simulink model "motor_kit_sim_20MHz"  (R2024a)
settings: Solver=VariableStepAuto  StartTime=0.0  StopTime=10*62.5E-6  RelTol=1e-3  EnableMultiTasking=on
PreLoadFcn:
  | setup_motor_kit_sim_20MHz;
InitFcn:
  | setup_motor_kit_sim_20MHz;
values from neighbouring files (symbols this model uses):
  DSPBASampleTime = 0.05e-6    (= 5e-08)    [setup_motor_kit_sim_20MHz.m]
  wordLength = 16    [setup_motor_kit_sim_20MHz.m]
undefined symbols (not defined in the file or in its folder): AdvDSPBChannelOutDisplay, dpoly, dspba_internal_get_channel_ports, evalAionMaskParam, latency, primtype, value, x
libraries: DSPBAPrim x317, DSPBAModelBus x25, DSPBABase x7, dspsrcs4 x3, simulink x3, DSPBAUtilities x1
(part 3 of 4)

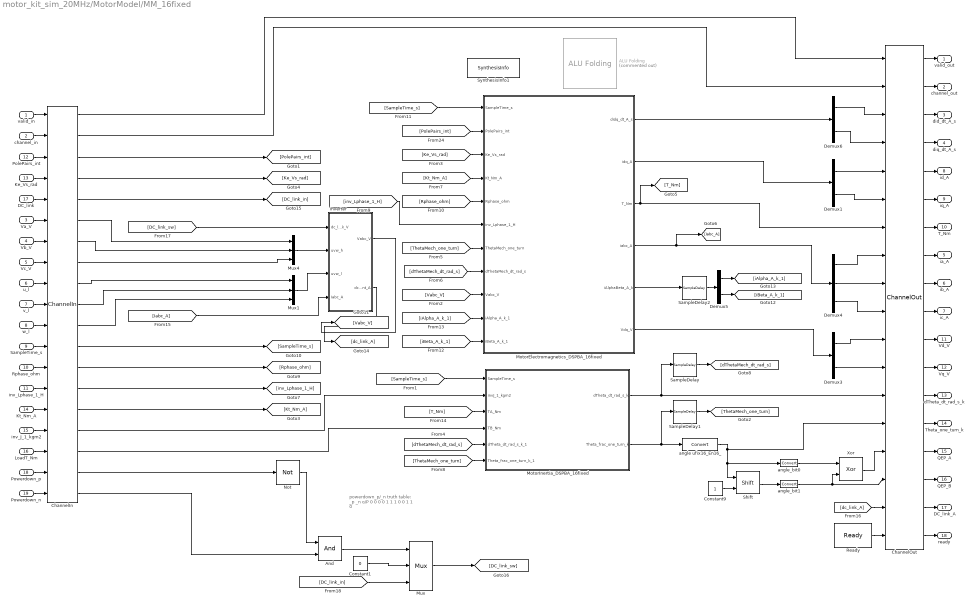
== system motor_kit_sim_20MHz/MotorModel/MM_16fixed ==
  note: powerdown_p/_n truth table:
      |
      | 	_p		_n		o/P
      | 	0		0		0
      | 	0		1		1
      | 	1		0		0
      | 	1		1		0
  valid_in : Inport
  channel_in : Inport  Port=2
  Va_V : Inport  Port=3
  Vb_V : Inport  Port=4
  Vc_V : Inport  Port=5
  u_l : Inport  Port=6  OutDataTypeStr=boolean
  v_l : Inport  Port=7  OutDataTypeStr=boolean
  w_l : Inport  Port=8  OutDataTypeStr=boolean
  SampleTime_s : Inport  Port=9
  Rphase_ohm : Inport  Port=10
  inv_Lphase_1_H : Inport  Port=11
  PolePairs_int : Inport  Port=12
  Ke_Vs_rad : Inport  Port=13
  Kt_Nm_A : Inport  Port=14
  inv_J_1_kgm2 : Inport  Port=15
  LoadT_Nm : Inport  Port=16
  DC_link : Inport  Port=17
  Powerdown_p : Inport  Port=18
  Powerdown_n : Inport  Port=19
  ALU Folding : DSPBAUtilities/ALU Folding  Description=Enables the new folder. When this block is placed in a subsystem, all primitive subsystems at the level it is placed and below will be passed to the folder. DSP Builder will then generate folded subsystems which can be placed back into the existing design.  Commented=on  version=20130913  genModelFileName=folded_model.xml  sampleRate=SampleRate  numChannels=1  maxLatency=LatencyConstraint  inputFormat=Parallel  outputFormat=Parallel  latchOutputs=off  originalRate=off  hasIdleState=off  padInputs=off  simRate=Data rate
  And : DSPBAPrim/And  primtype=and  nInputs=2  nOutputs=1  omode=Inherit via internal rule  otype=sfix(16)  scale=2^-15  rndmethod=Unbiased  factor=1  satmethod=Symmetric  shift_vec=[0 1 2 -1]  value=0  inPortNames=[' '; ' '; ' '; ' '; ' '; ' '; ' '; ' '; ' '; ' '; ' '; ' '; ' '; ' '; ' '; ' '; ]  outPortNames=[' ']  dspbaimage=dspba_prim.svg  text=fprintf('&');  version=20240716
  ChannelIn : DSPBAPrim/ChannelIn  primtype=channelin  nInputs=dspba_internal_get_channel_ports(gcb)  nOutputs=dspba_internal_get_channel_ports(gcb)  omode=Inherit via internal rule  otype=sfix(16)  scale=2^-15  rndmethod=Unbiased  factor=1  satmethod=Symmetric  shift_vec=[0 1 2 -1]  value=17  inPortNames=['v'; 'c'; '0'; '1'; '2'; '3'; '4'; '5'; '6'; '7'; '8'; '9'; 'A'; 'B'; 'D'; 'E'; 'F'; 'G'; 'H'; 'I'; 'J'; 'K'; 'L'; 'M'; 'N'; 'O'; 'P'; 'Q'; 'R'; 'S'; 'T'; 'U'; 'W'; 'X'; 'Y'; 'Z']  outPortNames=['v'; 'c'; '0'; '1'; '2'; '3'; '4'; '5'; '6'; '7'; '8'; '9'; 'A'; 'B'; 'D'; 'E'; 'F'; 'G'; 'H'; 'I'; 'J'; 'K'; 'L'; 'M'; 'N'; 'O'; 'P'; 'Q'; 'R'; 'S'; 'T'; 'U'; 'W'; 'X'; 'Y'; 'Z']  dspbaimage=dspba_prim_channel_tall.svg  text=fprintf('In');  dataSignals=17  foldingEnabled=off  packetBeginPresent=off  packetBeginEnabled=off  version=20231204
  ChannelOut : DSPBAPrim/ChannelOut  primtype=channelout  nInputs=dspba_internal_get_channel_ports(gcb)  nOutputs=dspba_internal_get_channel_ports(gcb)  omode=Inherit via internal rule  otype=sfix(16)  scale=2^-15  rndmethod=Unbiased  factor=1  satmethod=Symmetric  shift_vec=[0 1 2 -1]  value=16  inPortNames=['v'; 'c'; '0'; '1'; '2'; '3'; '4'; '5'; '6'; '7'; '8'; '9'; 'A'; 'B'; 'D'; 'E'; 'F'; 'G'; 'H'; 'I'; 'J'; 'K'; 'L'; 'M'; 'N'; 'O'; 'P'; 'Q'; 'R'; 'S'; 'T'; 'U'; 'W'; 'X'; 'Y'; 'Z']  outPortNames=['v'; 'c'; '0'; '1'; '2'; '3'; '4'; '5'; '6'; '7'; '8'; '9'; 'A'; 'B'; 'D'; 'E'; 'F'; 'G'; 'H'; 'I'; 'J'; 'K'; 'L'; 'M'; 'N'; 'O'; 'P'; 'Q'; 'R'; 'S'; 'T'; 'U'; 'W'; 'X'; 'Y'; 'Z']  dspbaimage=dspba_prim_channel_tall.svg  text=fprintf('Out%s', AdvDSPBChannelOutDisplay(latency));  dataSignals=16  foldingEnabled=off  packetBeginPresent=off  packetBeginEnabled=off  latency=53  version=20230901
  Constant1 : Constant  Value=0  OutDataTypeStr=fixdt(1,16,6)  SampleTime=DSPBASampleTime
  Constant9 : Constant  OutDataTypeStr=boolean
  Demux{1,3,5..6} (4 alike) : Demux  Outputs=2
  Demux4 : Demux  Outputs=3
  MotorElectromagnetics_DSPBA_16fixed : Subsystem
  MotorInertia_DSPBA_16fixed : Subsystem
  Mux : DSPBAPrim/Mux  primtype=mux  nInputs=evalAionMaskParam(gcb,'value',1)+1  nOutputs=1  omode=Inherit via internal rule  otype=sfix(16)  scale=2^-15  rndmethod=Unbiased  factor=1  satmethod=Symmetric  shift_vec=[0 1 2 -1]  value=2  inPortNames=['s '; 'd0'; 'd1'; 'd2'; 'd3'; 'd4'; 'd5'; 'd6'; 'd7'; 'd8'; 'd9';]  outPortNames=[' ']  dspbaimage=dspba_prim_tall.svg  text=fprintf('%s', primtype);  version=20240715
  Mux1 : Mux  Inputs=3
  Mux4 : Mux  Inputs=3
  Not : DSPBAPrim/Not  primtype=not  nInputs=1  nOutputs=1  omode=Inherit via internal rule  otype=sfix(16)  scale=2^-15  rndmethod=Unbiased  factor=1  satmethod=Symmetric  shift_vec=[0 1 2 -1]  value=0  inPortNames=[' '; ' ';]  outPortNames=[' ']  dspbaimage=dspba_prim.svg  text=fprintf('~');  version=20240716
  Ready : DSPBAPrim/Ready  primtype=ready  nInputs=0  nOutputs=1  omode=Inherit via internal rule  otype=ufix(1)  scale=2^-0  rndmethod=Unbiased  factor=1  satmethod=Asymmetric  shift_vec=[]  value=1  inPortNames=['']  outPortNames=[' ']  dspbaimage=dspba_prim.svg  text=fprintf('Ready');  version=20240719
  SampleDelay : DSPBAPrim/SampleDelay  primtype=sampdelay  nInputs=1  nOutputs=1  omode=Inherit via internal rule  otype=sfix(16)  scale=2^-15  floatPrecision=float32_m23  rndmethod=Unbiased  factor=1  satmethod=Symmetric  shift_vec=[0 1 2 -1]  value=25  inPortNames=[' '; ' ';]  outPortNames=[' ']  dspbaimage=dspba_prim.svg  text=dpoly(1, eye(1,value+1), 'z')  flexible=on  slackgroup=0  augmented=28  version=20240711  advOptions=[]
  SampleDelay1 : DSPBAPrim/SampleDelay  primtype=sampdelay  nInputs=1  nOutputs=1  omode=Inherit via internal rule  otype=sfix(16)  scale=2^-15  floatPrecision=float32_m23  rndmethod=Unbiased  factor=1  satmethod=Symmetric  shift_vec=[0 1 2 -1]  value=33  inPortNames=[' '; ' ';]  outPortNames=[' ']  dspbaimage=dspba_prim.svg  text=dpoly(1, eye(1,value+1), 'z')  flexible=on  slackgroup=0  augmented=28  version=20240711  advOptions=[]
  SampleDelay2 : DSPBAPrim/SampleDelay  primtype=sampdelay  nInputs=1  nOutputs=1  omode=Inherit via internal rule  otype=sfix(16)  scale=2^-15  floatPrecision=float32_m23  rndmethod=Unbiased  factor=1  satmethod=Symmetric  shift_vec=[0 1 2 -1]  value=1  inPortNames=[' '; ' ';]  outPortNames=[' ']  dspbaimage=dspba_prim.svg  text=dpoly(1, eye(1,value+1), 'z')  flexible=off  slackgroup=0  augmented=0  version=20240711  advOptions=[]
  Shift : DSPBAPrim/Shift  primtype=shift  nInputs=2  nOutputs=1  omode=Specify via dialog  otype=ufix(16)  scale=2^-16  rndmethod=Unbiased  factor=1  satmethod=Symmetric  shift_vec=[0 1 2 -1]  value=0  inPortNames=['a'; 'b';]  outPortNames=[' ']  dspbaimage=dspba_prim.svg  text=fprintf('a >> b');  version=20240716
  SynthesisInfo1 : DSPBAPrim/SynthesisInfo  primtype=synthinfo  nInputs=0  nOutputs=0  omode=Inherit via internal rule  otype=sfix(16)  scale=2^-15  rndmethod=Truncate  factor=1  satmethod=Symmetric  shift_vec=[0 1 2 -1]  value=99  inPortNames=[' '; ' ';]  outPortNames=[' ']  dspbaimage=dspba_prim_ctrl.jpg  text=fprintf('Style=%s', style);  style=Scheduled  constraintPair=None  constraintRelation=>  constraintLimit=2  modelRefSign=+  modelRef=''  showSchedule=off  simulationMode=Use Global Value  resetMinimization=Conditional - On for ChannelIn/Out only  version=20230821
  Xor : DSPBAPrim/Xor  primtype=xor  nInputs=2  nOutputs=1  omode=Inherit via internal rule  otype=sfix(16)  scale=2^-15  rndmethod=Unbiased  factor=1  satmethod=Symmetric  shift_vec=[0 1 2 -1]  value=0  inPortNames=[' '; ' '; ' '; ' '; ' '; ' '; ' '; ' '; ' '; ' '; ' '; ' '; ' '; ' '; ' '; ' '; ]  outPortNames=[' ']  dspbaimage=dspba_prim.svg  text=fprintf('^');  version=20240716
  angle ufix16_En16_ : DSPBAPrim/Convert  primtype=convert  nInputs=1  nOutputs=1  omode=Specify via dialog  otype=ufix(16)  scale=2^-16  floatPrecision=float32_m23  rndmethod=Unbiased  factor=1  satmethod=None  shift_vec=[0 1 2 -1]  value=round([0:255]/17)  inPortNames=[' '; ' ';]  outPortNames=[' '; 'c']  dspbaimage=dspba_prim_wide.svg  text=fprintf('convert');  clipdetect=off  advOptions=[]  version=20240711
  angle_bit0 : DSPBAPrim/Convert  primtype=convert  nInputs=1  nOutputs=1  omode=Specify via dialog  otype=ufix(1)  scale=2^-13  floatPrecision=float32_m23  rndmethod=Truncate  factor=1  satmethod=None  shift_vec=[0 1 2 -1]  value=round([0:255]/17)  inPortNames=[' '; ' ';]  outPortNames=[' '; 'c']  dspbaimage=dspba_prim_wide.svg  text=fprintf('convert');  clipdetect=off  advOptions=[]  version=20240711
  angle_bit1 : DSPBAPrim/Convert  primtype=convert  nInputs=1  nOutputs=1  omode=Specify via dialog  otype=ufix(1)  scale=2^-13  floatPrecision=float32_m23  rndmethod=Truncate  factor=1  satmethod=None  shift_vec=[0 1 2 -1]  value=round([0:255]/17)  inPortNames=[' '; ' ';]  outPortNames=[' '; 'c']  dspbaimage=dspba_prim_wide.svg  text=fprintf('convert');  clipdetect=off  advOptions=[]  version=20240711
  inverter : Subsystem
  valid_out : Outport
  channel_out : Outport  Port=2
  did_dt_A_s : Outport  Port=3
  diq_dt_A_s : Outport  Port=4
  ia_A : Outport  Port=5
  ib_A : Outport  Port=6
  ic_A : Outport  Port=7
  id_A : Outport  Port=8
  iq_A : Outport  Port=9
  T_Nm : Outport  Port=10
  Vd_V : Outport  Port=11
  Vq_V : Outport  Port=12
  dTheta_dt_rad_s_k : Outport  Port=13
  Theta_one_turn_k : Outport  Port=14
  QEP_A : Outport  Port=15
  QEP_B : Outport  Port=16
  DC_link_A : Outport  Port=17
  ready : Outport  Port=18
  wires:
  [SampleTime_s] -> MotorElectromagnetics_DSPBA_16fixed/1(SampleTime_s)
  [PolePairs_int] -> MotorElectromagnetics_DSPBA_16fixed/2(PolePairs_int)
  [Ke_Vs_rad] -> MotorElectromagnetics_DSPBA_16fixed/3(Ke_Vs_rad)
  [Kt_Nm_A] -> MotorElectromagnetics_DSPBA_16fixed/4(Kt_Nm_A)
  [Rphase_ohm] -> MotorElectromagnetics_DSPBA_16fixed/5(Rphase_ohm)
  [inv_Lphase_1_H] -> MotorElectromagnetics_DSPBA_16fixed/6(inv_Lphase_1_H)
  [Vabc_V] -> MotorElectromagnetics_DSPBA_16fixed/9(Vabc_V)
  [iAlpha_A_k_1] -> MotorElectromagnetics_DSPBA_16fixed/10(iAlpha_A_k_1)
  [iBeta_A_k_1] -> MotorElectromagnetics_DSPBA_16fixed/11(iBeta_A_k_1)
  MotorElectromagnetics_DSPBA_16fixed/1(didq_dt_A_s) -> Demux6/1
  MotorElectromagnetics_DSPBA_16fixed/2(idq_A) -> Demux1/1
  MotorElectromagnetics_DSPBA_16fixed/3(T_Nm) -> ChannelOut/7, [T_Nm]
  [SampleTime_s] -> MotorInertia_DSPBA_16fixed/1(SampleTime_s)
  [dThetaMech_dt_rad_s] -> MotorInertia_DSPBA_16fixed/5(dTheta_dt_rad_s_k_1)
  [ThetaMech_one_turn] -> MotorInertia_DSPBA_16fixed/6(Theta_frac_one_turn_k_1)
  [T_Nm] -> MotorInertia_DSPBA_16fixed/3(TA_Nm)
  valid_in/1 -> ChannelIn/1
  channel_in/1 -> ChannelIn/2
  PolePairs_int/1 -> ChannelIn/3
  ChannelOut/1 -> valid_out/1
  ChannelOut/3 -> did_dt_A_s/1
  ChannelOut/2 -> channel_out/1
  ChannelOut/4 -> diq_dt_A_s/1
  ChannelOut/5 -> id_A/1
  ChannelOut/6 -> iq_A/1
  ChannelOut/7 -> T_Nm/1
  ChannelOut/8 -> ia_A/1
  ChannelOut/9 -> ib_A/1
  ChannelOut/10 -> ic_A/1
  ChannelIn/1 -> ChannelOut/1
  ChannelIn/2 -> ChannelOut/2
  ChannelIn/3 -> [PolePairs_int]
  Demux6/1 -> ChannelOut/3
  Demux6/2 -> ChannelOut/4
  Demux1/1 -> ChannelOut/5
  Demux1/2 -> ChannelOut/6
  MotorElectromagnetics_DSPBA_16fixed/4(iabc_A) -> [Iabc_A], Demux4/1
  Demux4/1 -> ChannelOut/8
  Demux4/2 -> ChannelOut/9
  Demux4/3 -> ChannelOut/10
  MotorElectromagnetics_DSPBA_16fixed/5(iAlphaBeta_A_k) -> SampleDelay2/1
  MotorElectromagnetics_DSPBA_16fixed/6(Vdq_V) -> Demux3/1
  MotorInertia_DSPBA_16fixed/1(dTheta_dt_rad_s_k) -> SampleDelay/1, ChannelOut/13
  SampleDelay1/1 -> [ThetaMech_one_turn]
  [ThetaMech_one_turn] -> MotorElectromagnetics_DSPBA_16fixed/7(ThetaMech_one_turn)
  [dThetaMech_dt_rad_s] -> MotorElectromagnetics_DSPBA_16fixed/8(dThetaMech_dt_rad_s)
  SampleDelay/1 -> [dThetaMech_dt_rad_s]
  SampleDelay2/1 -> Demux5/1
  Demux5/1 -> [iAlpha_A_k_1]
  Demux5/2 -> [iBeta_A_k_1]
  Ke_Vs_rad/1 -> ChannelIn/4
  ChannelIn/8 -> Mux4/3
  ChannelIn/6 -> Mux4/1
  ChannelIn/4 -> [Ke_Vs_rad]
  ChannelIn/7 -> Mux4/2
  Demux3/1 -> ChannelOut/11
  Demux3/2 -> ChannelOut/12
  ChannelOut/11 -> Vd_V/1
  ChannelOut/12 -> Vq_V/1
  ChannelOut/13 -> dTheta_dt_rad_s_k/1
  ChannelOut/14 -> Theta_one_turn_k/1
  Vc_V/1 -> ChannelIn/8
  Vb_V/1 -> ChannelIn/7
  Va_V/1 -> ChannelIn/6
  DC_link/1 -> ChannelIn/5
  Constant9/1 -> Shift/2
  Xor/1 -> ChannelOut/15
  Shift/1 -> angle_bit1/1
  angle_bit1/1 -> ChannelOut/16, Xor/2
  MotorInertia_DSPBA_16fixed/2(Theta_frac_one_turn_k) -> angle ufix16_En16_/1, SampleDelay1/1
  angle_bit0/1 -> Xor/1
  ChannelOut/15 -> QEP_A/1
  ChannelOut/16 -> QEP_B/1
  angle ufix16_En16_/1 -> ChannelOut/14, Shift/1, angle_bit0/1
  ChannelIn/5 -> [DC_link_in]
  u_l/1 -> ChannelIn/9
  w_l/1 -> ChannelIn/11
  v_l/1 -> ChannelIn/10
  SampleTime_s/1 -> ChannelIn/12
  Rphase_ohm/1 -> ChannelIn/13
  inv_Lphase_1_H/1 -> ChannelIn/14
  Kt_Nm_A/1 -> ChannelIn/15
  inv_J_1_kgm2/1 -> ChannelIn/16
  LoadT_Nm/1 -> ChannelIn/17
  ChannelIn/17 -> MotorInertia_DSPBA_16fixed/4(TB_Nm)
  ChannelIn/16 -> MotorInertia_DSPBA_16fixed/2(invJ_1_kgm2)
  ChannelIn/12 -> [SampleTime_s]
  ChannelIn/13 -> [Rphase_ohm]
  ChannelIn/15 -> [Kt_Nm_A]
  ChannelIn/14 -> [inv_Lphase_1_H]
  Mux1/1 -> inverter/3(uvw_l)
  ChannelIn/9 -> Mux1/1
  ChannelIn/11 -> Mux1/3
  ChannelIn/10 -> Mux1/2
  Mux4/1 -> inverter/2(uvw_h)
  inverter/1(Vabc_V) -> [Vabc_V]
  [Iabc_A] -> inverter/4(Iabc_A)
  Ready/1 -> ChannelOut/18
  ChannelOut/17 -> DC_link_A/1
  ChannelOut/18 -> ready/1
  [dc_link_A] -> ChannelOut/17
  inverter/2(dc_link_current_A) -> [dc_link_A]
  [DC_link_sw] -> inverter/1(dc_link_V)
  [DC_link_in] -> Mux/3
  Mux/1 -> [DC_link_sw]
  Constant1/1 -> Mux/2
  Not/1 -> And/1
  And/1 -> Mux/1
  Powerdown_p/1 -> ChannelIn/18
  Powerdown_n/1 -> ChannelIn/19
  ChannelIn/18 -> Not/1
  ChannelIn/19 -> And/2

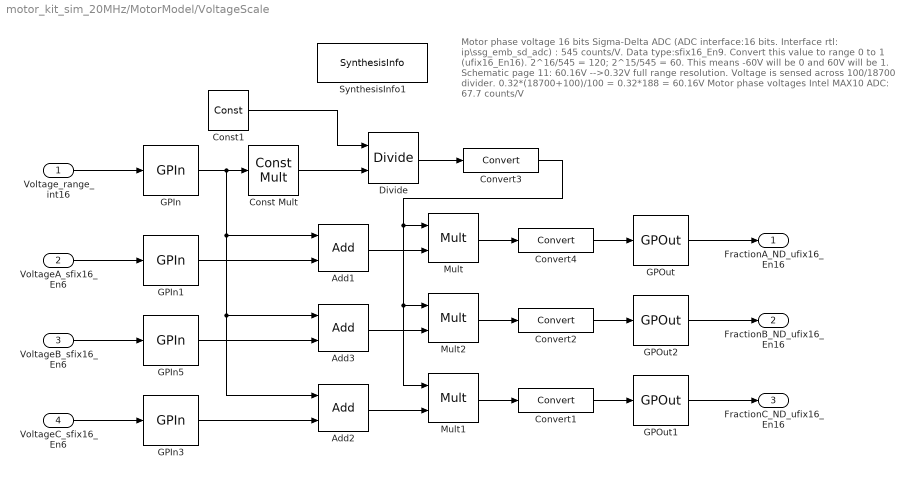
== system motor_kit_sim_20MHz/MotorModel/VoltageScale ==
  note: Motor phase voltage 16 bits Sigma-Delta ADC (ADC interface:16 bits. Interface rtl: ip\ssg_emb_sd_adc) : 545 counts/V. Data type:sfix16_En9. Convert this value to range 0 to 1 (ufix16_En16). 2^16/545 = 120; 2^15/545 = 60. This means -60V will be 0 and 60V will be 1.
      | Schematic page 11: 60.16V -->0.32V full range resolution. Voltage is sensed across 100/18700 divider. 0.32*(18700+100)/100 = 0.32*188 = 60.16V
      | Motor phase voltages Intel MAX10 ADC: 67.7 counts/V
  Voltage_range_int16 : Inport
  VoltageA_sfix16_En6 : Inport  Port=2
  VoltageB_sfix16_En6 : Inport  Port=3
  VoltageC_sfix16_En6 : Inport  Port=4
  Add1 : DSPBAPrim/Add  primtype=add  nInputs=evalAionMaskParam(gcb,'value',1)  nOutputs=1  omode=Inherit via internal rule with word growth  otype=sfix(16)  scale=2^-15  rndmethod=Unbiased  factor=1  satmethod=Symmetric  shift_vec=[0 1 2 -1]  value=2  inPortNames=[' '; ' ';]  outPortNames=[' ']  dspbaimage=dspba_prim.svg  text=fprintf('+');  genFPC=off  floatRounding=correct  advOptions=[]  version=20240716
  Add2 : DSPBAPrim/Add  primtype=add  nInputs=evalAionMaskParam(gcb,'value',1)  nOutputs=1  omode=Inherit via internal rule with word growth  otype=sfix(16)  scale=2^-15  rndmethod=Unbiased  factor=1  satmethod=Symmetric  shift_vec=[0 1 2 -1]  value=2  inPortNames=[' '; ' ';]  outPortNames=[' ']  dspbaimage=dspba_prim.svg  text=fprintf('+');  genFPC=off  floatRounding=correct  advOptions=[]  version=20240716
  Add3 : DSPBAPrim/Add  primtype=add  nInputs=evalAionMaskParam(gcb,'value',1)  nOutputs=1  omode=Inherit via internal rule with word growth  otype=sfix(16)  scale=2^-15  rndmethod=Unbiased  factor=1  satmethod=Symmetric  shift_vec=[0 1 2 -1]  value=2  inPortNames=[' '; ' ';]  outPortNames=[' ']  dspbaimage=dspba_prim.svg  text=fprintf('+');  genFPC=off  floatRounding=correct  advOptions=[]  version=20240716
  Const Mult : DSPBAPrim/Const Mult  primtype=constmult  nInputs=1  nOutputs=1  omode=Inherit via internal rule  otype=sfix(16)  scale=2^-15  rndmethod=Unbiased  factor=1  satmethod=Symmetric  shift_vec=[0 1 2 -1]  value=2  inPortNames=[' '; ' ';]  outPortNames=[' ']  dspbaimage=dspba_prim.svg  text=fprintf('cx');  floatRounding=correct  advOptions=[]  version=20240716
  Const1 : DSPBAPrim/Const  primtype=const  nInputs=0  nOutputs=1  omode=Specify via dialog  otype=sfix(2)  scale=1  floatPrecision=float32_m23  rndmethod=Unbiased  factor=1  satmethod=Symmetric  shift_vec=[0 1 2 -1]  value=1  inPortNames=['+'; '+';]  outPortNames=[' ']  dspbaimage=dspba_prim.svg  text=fprintf('%s', num2str(value));  warnSaturation=on  version=20240711  SampleTime=inf
  Convert1 : DSPBAPrim/Convert  primtype=convert  nInputs=1  nOutputs=1  omode=Specify via dialog  otype=DataTypeFraction  scale=constScaleFraction  floatPrecision=float32_m23  rndmethod=Biased  factor=1  satmethod=None  shift_vec=[0 1 2 -1]  value=round([0:255]/17)  inPortNames=[' '; ' ';]  outPortNames=[' '; 'c']  dspbaimage=dspba_prim_wide.svg  text=fprintf('convert');  clipdetect=off  advOptions=[]  version=20240711
  Convert2 : DSPBAPrim/Convert  primtype=convert  nInputs=1  nOutputs=1  omode=Specify via dialog  otype=DataTypeFraction  scale=constScaleFraction  floatPrecision=float32_m23  rndmethod=Biased  factor=1  satmethod=None  shift_vec=[0 1 2 -1]  value=round([0:255]/17)  inPortNames=[' '; ' ';]  outPortNames=[' '; 'c']  dspbaimage=dspba_prim_wide.svg  text=fprintf('convert');  clipdetect=off  advOptions=[]  version=20240711
  Convert3 : DSPBAPrim/Convert  primtype=convert  nInputs=1  nOutputs=1  omode=Specify via dialog  otype=sfix(18)  scale=constScaleFraction  floatPrecision=float32_m23  rndmethod=Biased  factor=1  satmethod=None  shift_vec=[0 1 2 -1]  value=round([0:255]/17)  inPortNames=[' '; ' ';]  outPortNames=[' '; 'c']  dspbaimage=dspba_prim_wide.svg  text=fprintf('convert');  clipdetect=off  advOptions=[]  version=20240711
  Convert4 : DSPBAPrim/Convert  primtype=convert  nInputs=1  nOutputs=1  omode=Specify via dialog  otype=DataTypeFraction  scale=constScaleFraction  floatPrecision=float32_m23  rndmethod=Biased  factor=1  satmethod=None  shift_vec=[0 1 2 -1]  value=round([0:255]/17)  inPortNames=[' '; ' ';]  outPortNames=[' '; 'c']  dspbaimage=dspba_prim_wide.svg  text=fprintf('convert');  clipdetect=off  advOptions=[]  version=20240711
  Divide : DSPBAPrim/Divide  primtype=divide  nInputs=2  nOutputs=1  omode=Inherit via internal rule  otype=sfix(16)  scale=2^-15  rndmethod=Unbiased  factor=1  satmethod=Symmetric  shift_vec=[0 1 2 -1]  value=round([0:255]/17)  inPortNames=[' '; ' ';]  outPortNames=[' ']  dspbaimage=dspba_prim.svg  text=fprintf('a\n----\nb');  floatRounding=correct  intDivider=off  advOptions=[]  version=20240716
  GPIn{,1,3,5} (4 alike) : DSPBAPrim/GPIn  primtype=gpin  nInputs=evalAionMaskParam(gcb,'value',1)  nOutputs=evalAionMaskParam(gcb,'value',1)  omode=Inherit via internal rule  otype=sfix(16)  scale=2^-15  rndmethod=Unbiased  factor=1  satmethod=Symmetric  shift_vec=[0 1 2 -1]  value=1  inPortNames=[' ' ' ' ' ' ' ' ' ' ' ' ' ' ' ' ' ' ' ' ' ' ' ' ' ' ' ' ' ' ' ' ' ' ' ' ' ' ' ' ' ' ' ' ' ' ' ' ' ' ' ' ' ' ' ' ' ' ' ' ' ' ' ' ' ' ' ' ' ']'  outPortNames=[' ' ' ' ' ' ' ' ' ' ' ' ' ' ' ' ' ' ' ' ' ' ' ' ' ' ' ' ' ' ' ' ' ' ' ' ' ' ' ' ' ' ' ' ' ' ' ' ' ' ' ' ' ' ' ' ' ' ' ' ' ' ' ' ' ' ' ' ' ']'  dspbaimage=dspba_prim_channel_tall.svg  text=fprintf('GPIn');  version=20231204
  GPOut : DSPBAPrim/GPOut  primtype=gpout  nInputs=evalAionMaskParam(gcb,'value',1)  nOutputs=evalAionMaskParam(gcb,'value',1)  omode=Inherit via internal rule  otype=sfix(16)  scale=2^-15  rndmethod=Unbiased  factor=1  satmethod=Symmetric  shift_vec=[0 1 2 -1]  value=1  inPortNames=[' ' ' ' ' ' ' ' ' ' ' ' ' ' ' ' ' ' ' ' ' ' ' ' ' ' ' ' ' ' ' ' ' ' ' ' ' ' ' ' ' ' ' ' ' ' ' ' ' ' ' ' ' ' ' ' ' ' ' ' ' ' ' ' ' ' ' ' ' ']'  outPortNames=[' ' ' ' ' ' ' ' ' ' ' ' ' ' ' ' ' ' ' ' ' ' ' ' ' ' ' ' ' ' ' ' ' ' ' ' ' ' ' ' ' ' ' ' ' ' ' ' ' ' ' ' ' ' ' ' ' ' ' ' ' ' ' ' ' ' ' ' ' ']'  dspbaimage=dspba_prim_channel_tall.svg  text=fprintf('GPOut');  latency=21  version=20230904
  GPOut1 : DSPBAPrim/GPOut  primtype=gpout  nInputs=evalAionMaskParam(gcb,'value',1)  nOutputs=evalAionMaskParam(gcb,'value',1)  omode=Inherit via internal rule  otype=sfix(16)  scale=2^-15  rndmethod=Unbiased  factor=1  satmethod=Symmetric  shift_vec=[0 1 2 -1]  value=1  inPortNames=[' ' ' ' ' ' ' ' ' ' ' ' ' ' ' ' ' ' ' ' ' ' ' ' ' ' ' ' ' ' ' ' ' ' ' ' ' ' ' ' ' ' ' ' ' ' ' ' ' ' ' ' ' ' ' ' ' ' ' ' ' ' ' ' ' ' ' ' ' ']'  outPortNames=[' ' ' ' ' ' ' ' ' ' ' ' ' ' ' ' ' ' ' ' ' ' ' ' ' ' ' ' ' ' ' ' ' ' ' ' ' ' ' ' ' ' ' ' ' ' ' ' ' ' ' ' ' ' ' ' ' ' ' ' ' ' ' ' ' ' ' ' ' ']'  dspbaimage=dspba_prim_channel_tall.svg  text=fprintf('GPOut');  latency=21  version=20230904
  GPOut2 : DSPBAPrim/GPOut  primtype=gpout  nInputs=evalAionMaskParam(gcb,'value',1)  nOutputs=evalAionMaskParam(gcb,'value',1)  omode=Inherit via internal rule  otype=sfix(16)  scale=2^-15  rndmethod=Unbiased  factor=1  satmethod=Symmetric  shift_vec=[0 1 2 -1]  value=1  inPortNames=[' ' ' ' ' ' ' ' ' ' ' ' ' ' ' ' ' ' ' ' ' ' ' ' ' ' ' ' ' ' ' ' ' ' ' ' ' ' ' ' ' ' ' ' ' ' ' ' ' ' ' ' ' ' ' ' ' ' ' ' ' ' ' ' ' ' ' ' ' ']'  outPortNames=[' ' ' ' ' ' ' ' ' ' ' ' ' ' ' ' ' ' ' ' ' ' ' ' ' ' ' ' ' ' ' ' ' ' ' ' ' ' ' ' ' ' ' ' ' ' ' ' ' ' ' ' ' ' ' ' ' ' ' ' ' ' ' ' ' ' ' ' ' ']'  dspbaimage=dspba_prim_channel_tall.svg  text=fprintf('GPOut');  latency=21  version=20230904
  Mult : DSPBAPrim/Mult  primtype=mult  nInputs=2  nOutputs=1  omode=Inherit via internal rule  otype=sfix(16)  scale=2^-15  floatPrecision=float32_m23  rndmethod=Unbiased  factor=1  satmethod=Symmetric  shift_vec=[0 1 2 -1]  value=0  inPortNames=[' '; ' ';]  outPortNames=[' ']  dspbaimage=dspba_prim.svg  text=fprintf('X');  floatRounding=correct  advOptions=[]  version=20240711
  Mult1 : DSPBAPrim/Mult  primtype=mult  nInputs=2  nOutputs=1  omode=Inherit via internal rule  otype=sfix(16)  scale=2^-15  floatPrecision=float32_m23  rndmethod=Unbiased  factor=1  satmethod=Symmetric  shift_vec=[0 1 2 -1]  value=0  inPortNames=[' '; ' ';]  outPortNames=[' ']  dspbaimage=dspba_prim.svg  text=fprintf('X');  floatRounding=correct  advOptions=[]  version=20240711
  Mult2 : DSPBAPrim/Mult  primtype=mult  nInputs=2  nOutputs=1  omode=Inherit via internal rule  otype=sfix(16)  scale=2^-15  floatPrecision=float32_m23  rndmethod=Unbiased  factor=1  satmethod=Symmetric  shift_vec=[0 1 2 -1]  value=0  inPortNames=[' '; ' ';]  outPortNames=[' ']  dspbaimage=dspba_prim.svg  text=fprintf('X');  floatRounding=correct  advOptions=[]  version=20240711
  SynthesisInfo1 : DSPBAPrim/SynthesisInfo  primtype=synthinfo  nInputs=0  nOutputs=0  omode=Inherit via internal rule  otype=sfix(16)  scale=2^-15  rndmethod=Truncate  factor=1  satmethod=Symmetric  shift_vec=[0 1 2 -1]  value=99  inPortNames=[' '; ' ';]  outPortNames=[' ']  dspbaimage=dspba_prim_ctrl.jpg  text=fprintf('Style=%s', style);  style=Scheduled  constraintPair=None  constraintRelation=>  constraintLimit=2  modelRefSign=+  modelRef=''  showSchedule=off  simulationMode=Use Global Value  resetMinimization=Conditional - On for ChannelIn/Out only  version=20230821
  "FractionA_ND_ufix16_En16 " : Outport
  FractionB_ND_ufix16_En16 : Outport  Port=2
  FractionC_ND_ufix16_En16 : Outport  Port=3
  wires:
  GPOut2/1 -> FractionB_ND_ufix16_En16/1
  GPOut1/1 -> FractionC_ND_ufix16_En16/1
  Convert2/1 -> GPOut2/1
  Convert1/1 -> GPOut1/1
  Mult1/1 -> Convert1/1
  Mult/1 -> Convert4/1
  Const1/1 -> Divide/1
  VoltageC_sfix16_En6/1 -> GPIn3/1
  Mult2/1 -> Convert2/1
  Voltage_range_int16/1 -> GPIn/1
  VoltageB_sfix16_En6/1 -> GPIn5/1
  GPOut/1 -> "FractionA_ND_ufix16_En16 "/1
  GPIn/1 -> Const Mult/1, Add1/1, Add3/1, Add2/1
  GPIn3/1 -> Add2/2
  Convert4/1 -> GPOut/1
  GPIn5/1 -> Add3/2
  VoltageA_sfix16_En6/1 -> GPIn1/1
  Add2/1 -> Mult1/2
  Add3/1 -> Mult2/2
  Add1/1 -> Mult/2
  GPIn1/1 -> Add1/2
  Const Mult/1 -> Divide/2
  Divide/1 -> Convert3/1
  Convert3/1 -> Mult1/1, Mult2/1, Mult/1

== system motor_kit_sim_20MHz/MotorModel/Voltage_scale_120_link_V ==
  note: DC link voltage 16 bits Sigma-Delta ADC (ADC interface:16 bits. Interface rtl: ip\dspba\two_phase_dc_dc\rtl\psg_ecfs_lvdcdc_sd_adc\hdl) : 545 counts/V. Data type:sfix16_En9. Convert this value to range 0 to 1 (ufix16_En16). 2^16/545 = 120; 2^15/545 = 60. This means -60V will be 0 and 60V will be 1.
      | Schematic page 6: 60.16V -->0.32V full range resolution. Voltage is sensed across 100/18700 divider. 0.32*(18700+100)/100=60.16V
      | This voltage has been scaled differently to be feedback into DC-DC controller IP.
      | Scaling for DC-DC controller IP input voltage_fdbk: 40 counts/V. This scaling is handled within ip\dspba\two_phase_dc_dc\rtl\psg_ecfs_lvdcdc_sd_adc\hdl\psg_ecfs_lvdcdc_sd_adc.v, it is scaled in hardware.
      | DC link voltage Intel MAX10 ADC: 67.7 counts/V
  Voltage_range_int16 : Inport
  Voltage_sfix16_En9 : Inport  Port=2
  Add1 : DSPBAPrim/Add  primtype=add  nInputs=evalAionMaskParam(gcb,'value',1)  nOutputs=1  omode=Inherit via internal rule with word growth  otype=sfix(16)  scale=2^-15  rndmethod=Unbiased  factor=1  satmethod=Symmetric  shift_vec=[0 1 2 -1]  value=2  inPortNames=[' '; ' ';]  outPortNames=[' ']  dspbaimage=dspba_prim.svg  text=fprintf('+');  genFPC=off  floatRounding=correct  advOptions=[]  version=20240716
  Const2 : DSPBAPrim/Const  primtype=const  nInputs=0  nOutputs=1  omode=Specify via dialog  otype=DataType  scale=constScaleFraction  floatPrecision=float32_m23  rndmethod=Unbiased  factor=1  satmethod=Symmetric  shift_vec=[0 1 2 -1]  value=1/2  inPortNames=['+'; '+';]  outPortNames=[' ']  dspbaimage=dspba_prim.svg  text=fprintf('%s', num2str(value));  warnSaturation=on  version=20240711  SampleTime=inf
  Convert4 : DSPBAPrim/Convert  primtype=convert  nInputs=1  nOutputs=1  omode=Specify via dialog  otype=DataTypeFraction  scale=constScaleFraction  floatPrecision=float32_m23  rndmethod=Biased  factor=1  satmethod=None  shift_vec=[0 1 2 -1]  value=round([0:255]/17)  inPortNames=[' '; ' ';]  outPortNames=[' '; 'c']  dspbaimage=dspba_prim_wide.svg  text=fprintf('convert');  clipdetect=off  advOptions=[]  version=20240711
  Divide : DSPBAPrim/Divide  primtype=divide  nInputs=2  nOutputs=1  omode=Inherit via internal rule  otype=sfix(16)  scale=2^-15  rndmethod=Unbiased  factor=1  satmethod=Symmetric  shift_vec=[0 1 2 -1]  value=round([0:255]/17)  inPortNames=[' '; ' ';]  outPortNames=[' ']  dspbaimage=dspba_prim.svg  text=fprintf('a\n----\nb');  floatRounding=correct  intDivider=off  advOptions=[]  version=20240716
  GPIn : DSPBAPrim/GPIn  primtype=gpin  nInputs=evalAionMaskParam(gcb,'value',1)  nOutputs=evalAionMaskParam(gcb,'value',1)  omode=Inherit via internal rule  otype=sfix(16)  scale=2^-15  rndmethod=Unbiased  factor=1  satmethod=Symmetric  shift_vec=[0 1 2 -1]  value=1  inPortNames=[' ' ' ' ' ' ' ' ' ' ' ' ' ' ' ' ' ' ' ' ' ' ' ' ' ' ' ' ' ' ' ' ' ' ' ' ' ' ' ' ' ' ' ' ' ' ' ' ' ' ' ' ' ' ' ' ' ' ' ' ' ' ' ' ' ' ' ' ' ']'  outPortNames=[' ' ' ' ' ' ' ' ' ' ' ' ' ' ' ' ' ' ' ' ' ' ' ' ' ' ' ' ' ' ' ' ' ' ' ' ' ' ' ' ' ' ' ' ' ' ' ' ' ' ' ' ' ' ' ' ' ' ' ' ' ' ' ' ' ' ' ' ' ']'  dspbaimage=dspba_prim_channel_tall.svg  text=fprintf('GPIn');  version=20231204
  GPIn1 : DSPBAPrim/GPIn  primtype=gpin  nInputs=evalAionMaskParam(gcb,'value',1)  nOutputs=evalAionMaskParam(gcb,'value',1)  omode=Inherit via internal rule  otype=sfix(16)  scale=2^-15  rndmethod=Unbiased  factor=1  satmethod=Symmetric  shift_vec=[0 1 2 -1]  value=1  inPortNames=[' ' ' ' ' ' ' ' ' ' ' ' ' ' ' ' ' ' ' ' ' ' ' ' ' ' ' ' ' ' ' ' ' ' ' ' ' ' ' ' ' ' ' ' ' ' ' ' ' ' ' ' ' ' ' ' ' ' ' ' ' ' ' ' ' ' ' ' ' ']'  outPortNames=[' ' ' ' ' ' ' ' ' ' ' ' ' ' ' ' ' ' ' ' ' ' ' ' ' ' ' ' ' ' ' ' ' ' ' ' ' ' ' ' ' ' ' ' ' ' ' ' ' ' ' ' ' ' ' ' ' ' ' ' ' ' ' ' ' ' ' ' ' ']'  dspbaimage=dspba_prim_channel_tall.svg  text=fprintf('GPIn');  version=20231204
  GPOut : DSPBAPrim/GPOut  primtype=gpout  nInputs=evalAionMaskParam(gcb,'value',1)  nOutputs=evalAionMaskParam(gcb,'value',1)  omode=Inherit via internal rule  otype=sfix(16)  scale=2^-15  rndmethod=Unbiased  factor=1  satmethod=Symmetric  shift_vec=[0 1 2 -1]  value=1  inPortNames=[' ' ' ' ' ' ' ' ' ' ' ' ' ' ' ' ' ' ' ' ' ' ' ' ' ' ' ' ' ' ' ' ' ' ' ' ' ' ' ' ' ' ' ' ' ' ' ' ' ' ' ' ' ' ' ' ' ' ' ' ' ' ' ' ' ' ' ' ' ']'  outPortNames=[' ' ' ' ' ' ' ' ' ' ' ' ' ' ' ' ' ' ' ' ' ' ' ' ' ' ' ' ' ' ' ' ' ' ' ' ' ' ' ' ' ' ' ' ' ' ' ' ' ' ' ' ' ' ' ' ' ' ' ' ' ' ' ' ' ' ' ' ' ']'  dspbaimage=dspba_prim_channel_tall.svg  text=fprintf('GPOut');  latency=28  version=20230904
  Mult : DSPBAPrim/Mult  primtype=mult  nInputs=2  nOutputs=1  omode=Inherit via internal rule  otype=sfix(16)  scale=2^-15  floatPrecision=float32_m23  rndmethod=Unbiased  factor=1  satmethod=Symmetric  shift_vec=[0 1 2 -1]  value=0  inPortNames=[' '; ' ';]  outPortNames=[' ']  dspbaimage=dspba_prim.svg  text=fprintf('X');  floatRounding=correct  advOptions=[]  version=20240711
  SynthesisInfo1 : DSPBAPrim/SynthesisInfo  primtype=synthinfo  nInputs=0  nOutputs=0  omode=Inherit via internal rule  otype=sfix(16)  scale=2^-15  rndmethod=Truncate  factor=1  satmethod=Symmetric  shift_vec=[0 1 2 -1]  value=99  inPortNames=[' '; ' ';]  outPortNames=[' ']  dspbaimage=dspba_prim_ctrl.jpg  text=fprintf('Style=%s', style);  style=Scheduled  constraintPair=None  constraintRelation=>  constraintLimit=2  modelRefSign=+  modelRef=''  showSchedule=off  simulationMode=Use Global Value  resetMinimization=Conditional - On for ChannelIn/Out only  version=20230821
  "Fraction_ND_ufix16_En16 " : Outport
  wires:
  Mult/1 -> Convert4/1
  GPIn/1 -> Add1/2
  GPIn1/1 -> Add1/1, Divide/2
  Voltage_sfix16_En9/1 -> GPIn/1
  Add1/1 -> Mult/2
  Convert4/1 -> GPOut/1
  GPOut/1 -> "Fraction_ND_ufix16_En16 "/1
  Voltage_range_int16/1 -> GPIn1/1
  Const2/1 -> Divide/1
  Divide/1 -> Mult/1

== system motor_kit_sim_20MHz/Output Filtering and Scaling/Sinc3 Filter ==
  In1 : Inport
  Add3 : Sum  Inputs=+-
  Constant2 : Constant  Value=60
  Discrete Filter2 : DiscreteFilter  Denominator=[1 -1]
  Discrete Filter3 : DiscreteFilter  Denominator=[1 -1]
  Discrete Filter4 : DiscreteFilter  Denominator=[1 -1]
  Discrete Filter5 : DiscreteFilter  Numerator=[1 -1]  Denominator=[1]
  Discrete Filter6 : DiscreteFilter  Numerator=[1 -1]  Denominator=[1]
  Discrete Filter8 : DiscreteFilter  Numerator=[1 -1]  Denominator=[1]
  Gain : Gain  Gain=1/128
  Gain4 : Gain  Gain=1/128
  Gain5 : Gain  Gain=1/128
  Gain6 : Gain  Gain=120
  Zero-Order Hold : ZeroOrderHold  SampleTime=128*DSPBASampleTime
  Out1 : Outport
  wires:
  Gain4/1 -> Discrete Filter6/1
  Gain/1 -> Discrete Filter8/1
  Discrete Filter2/1 -> Discrete Filter3/1
  Discrete Filter3/1 -> Discrete Filter4/1
  Gain5/1 -> Gain6/1
  Gain6/1 -> Add3/1
  Discrete Filter8/1 -> Gain4/1
  Discrete Filter4/1 -> Zero-Order Hold/1
  Zero-Order Hold/1 -> Discrete Filter5/1
  Constant2/1 -> Add3/2
  Discrete Filter6/1 -> Gain5/1
  Discrete Filter5/1 -> Gain/1
  Add3/1 -> Out1/1
  In1/1 -> Discrete Filter2/1

== system motor_kit_sim_20MHz/Output Filtering and Scaling/Sinc3 Filter1 ==
  In1 : Inport
  Add3 : Sum  Inputs=+-
  Constant2 : Constant  Value=32
  Discrete Filter2 : DiscreteFilter  Denominator=[1 -1]
  Discrete Filter3 : DiscreteFilter  Denominator=[1 -1]
  Discrete Filter4 : DiscreteFilter  Denominator=[1 -1]
  Discrete Filter5 : DiscreteFilter  Numerator=[1 -1]  Denominator=[1]
  Discrete Filter6 : DiscreteFilter  Numerator=[1 -1]  Denominator=[1]
  Discrete Filter8 : DiscreteFilter  Numerator=[1 -1]  Denominator=[1]
  Gain : Gain  Gain=1/128
  Gain4 : Gain  Gain=1/128
  Gain5 : Gain  Gain=1/128
  Gain6 : Gain  Gain=64
  Zero-Order Hold : ZeroOrderHold  SampleTime=128*DSPBASampleTime
  Out1 : Outport
  wires:
  Gain4/1 -> Discrete Filter6/1
  Gain/1 -> Discrete Filter8/1
  Discrete Filter2/1 -> Discrete Filter3/1
  Discrete Filter3/1 -> Discrete Filter4/1
  Gain5/1 -> Gain6/1
  Gain6/1 -> Add3/1
  Discrete Filter8/1 -> Gain4/1
  Discrete Filter4/1 -> Zero-Order Hold/1
  Zero-Order Hold/1 -> Discrete Filter5/1
  Constant2/1 -> Add3/2
  Discrete Filter6/1 -> Gain5/1
  Discrete Filter5/1 -> Gain/1
  Add3/1 -> Out1/1
  In1/1 -> Discrete Filter2/1

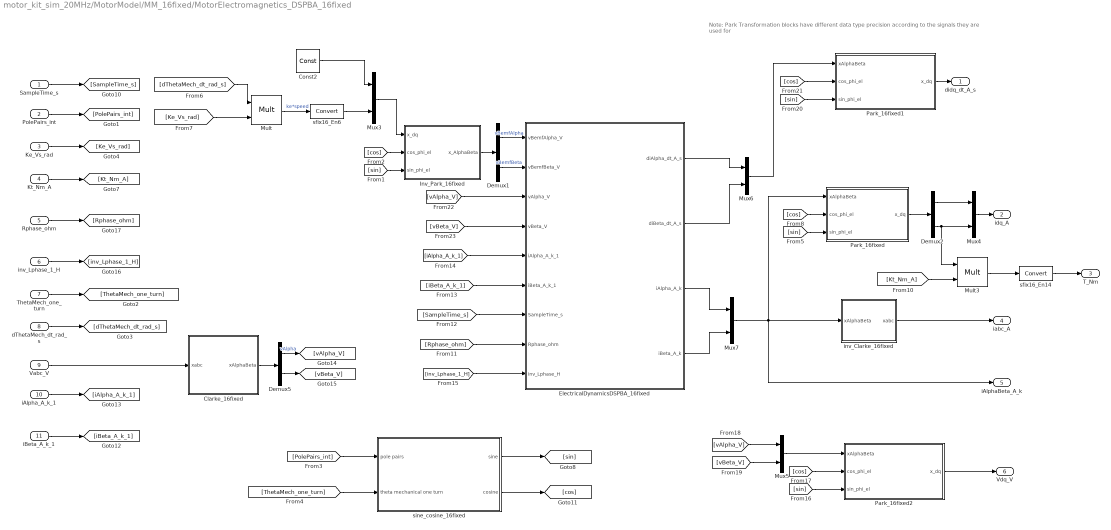
== system motor_kit_sim_20MHz/MotorModel/MM_16fixed/MotorElectromagnetics_DSPBA_16fixed ==
  note: Note: Park Transformation blocks have different data type precision according to the signals they are used for
  SampleTime_s : Inport
  PolePairs_int : Inport  Port=2
  Ke_Vs_rad : Inport  Port=3
  Kt_Nm_A : Inport  Port=4
  Rphase_ohm : Inport  Port=5
  inv_Lphase_1_H : Inport  Port=6
  ThetaMech_one_turn : Inport  Port=7
  dThetaMech_dt_rad_s : Inport  Port=8
  Vabc_V : Inport  Port=9
  iAlpha_A_k_1 : Inport  Port=10
  iBeta_A_k_1 : Inport  Port=11
  Clarke_16fixed : Subsystem
  Const2 : DSPBAPrim/Const  primtype=const  nInputs=0  nOutputs=1  omode=Specify via dialog  otype=DataType  scale=constScaleVoltage  floatPrecision=float32_m23  rndmethod=Unbiased  factor=1  satmethod=Symmetric  shift_vec=[0 1 2 -1]  value=0  inPortNames=['+'; '+';]  outPortNames=[' ']  dspbaimage=dspba_prim.svg  text=fprintf('%s', num2str(value));  warnSaturation=on  version=20240711  SampleTime=inf
  Demux1 : Demux  Outputs=2
  Demux2 : Demux  Outputs=2
  Demux5 : Demux  Outputs=2
  ElectricalDynamicsDSPBA_16fixed : Subsystem
  Inv_Park_16fixed : Subsystem
  Mult : DSPBAPrim/Mult  primtype=mult  nInputs=2  nOutputs=1  omode=Inherit via internal rule  otype=DataType  scale=constScaleVoltage  floatPrecision=float32_m23  rndmethod=Unbiased  factor=1  satmethod=Symmetric  shift_vec=[0 1 2 -1]  value=0  inPortNames=[' '; ' ';]  outPortNames=[' ']  dspbaimage=dspba_prim.svg  text=fprintf('X');  floatRounding=correct  advOptions=[]  version=20240711
  Mult3 : DSPBAPrim/Mult  primtype=mult  nInputs=2  nOutputs=1  omode=Inherit via internal rule  otype=DataType  scale=constScaleTorque  floatPrecision=float32_m23  rndmethod=Unbiased  factor=1  satmethod=Symmetric  shift_vec=[0 1 2 -1]  value=0  inPortNames=[' '; ' ';]  outPortNames=[' ']  dspbaimage=dspba_prim.svg  text=fprintf('X');  floatRounding=correct  advOptions=[]  version=20240711
  Mux{3..7} (5 alike) : Mux  Inputs=2
  Park_16fixed : Subsystem
  Park_16fixed1 : Subsystem
  Park_16fixed2 : Subsystem
  inv_Clarke_16fixed : Subsystem
  sfix16_En14 : DSPBAPrim/Convert  primtype=convert  nInputs=1  nOutputs=1  omode=Specify via dialog  otype=DataTypeTorque  scale=constScaleTorque  floatPrecision=float32_m23  rndmethod=Unbiased  factor=1  satmethod=Symmetric  shift_vec=[0 1 2 -1]  value=round([0:255]/17)  inPortNames=[' '; ' ';]  outPortNames=[' '; 'c']  dspbaimage=dspba_prim_wide.svg  text=fprintf('convert');  clipdetect=off  advOptions=[]  version=20240711
  sfix16_En6 : DSPBAPrim/Convert  primtype=convert  nInputs=1  nOutputs=1  omode=Specify via dialog  otype=DataType  scale=constScaleVoltage  floatPrecision=float32_m23  rndmethod=Unbiased  factor=1  satmethod=Symmetric  shift_vec=[0 1 2 -1]  value=round([0:255]/17)  inPortNames=[' '; ' ';]  outPortNames=[' '; 'c']  dspbaimage=dspba_prim_wide.svg  text=fprintf('convert');  clipdetect=off  advOptions=[]  version=20240711
  sine_cosine_16fixed : Subsystem
  didq_dt_A_s : Outport
  idq_A : Outport  Port=2
  T_Nm : Outport  Port=3
  iabc_A : Outport  Port=4
  iAlphaBeta_A_k : Outport  Port=5
  Vdq_V : Outport  Port=6
  wires:
  Mult3/1 -> sfix16_En14/1
  [Kt_Nm_A] -> Mult3/2
  sine_cosine_16fixed/2(cosine) -> [cos]
  sine_cosine_16fixed/1(sine) -> [sin]
  [ThetaMech_one_turn] -> sine_cosine_16fixed/2(theta mechanical one turn)
  [PolePairs_int] -> sine_cosine_16fixed/1(pole pairs)
  Park_16fixed2/1(x_dq) -> Vdq_V/1
  [sin] -> Park_16fixed2/3(sin_phi_el)
  [cos] -> Park_16fixed2/2(cos_phi_el)
  Mux5/1 -> Park_16fixed2/1(xAlphaBeta)
  [vAlpha_V] -> Mux5/1
  [vBeta_V] -> Mux5/2
  inv_Clarke_16fixed/1(xabc) -> iabc_A/1
  Mux7/1 -> iAlphaBeta_A_k/1, Park_16fixed/1(xAlphaBeta), inv_Clarke_16fixed/1(xAlphaBeta)
  Mux4/1 -> idq_A/1
  Demux2/2 -> Mux4/2, Mult3/1
  Demux2/1 -> Mux4/1
  [sin] -> Park_16fixed/3(sin_phi_el)
  [cos] -> Park_16fixed/2(cos_phi_el)
  Park_16fixed/1(x_dq) -> Demux2/1
  Park_16fixed1/1(x_dq) -> didq_dt_A_s/1
  ElectricalDynamicsDSPBA_16fixed/2(diBeta_dt_A_s) -> Mux6/2
  ElectricalDynamicsDSPBA_16fixed/1(diAlpha_dt_A_s) -> Mux6/1
  [sin] -> Inv_Park_16fixed/3(sin_phi_el)
  [cos] -> Inv_Park_16fixed/2(cos_phi_el)
  [cos] -> Park_16fixed1/2(cos_phi_el)
  Mux6/1 -> Park_16fixed1/1(xAlphaBeta)
  [sin] -> Park_16fixed1/3(sin_phi_el)
  [inv_Lphase_1_H] -> ElectricalDynamicsDSPBA_16fixed/9(inv_Lphase_H)
  [Rphase_ohm] -> ElectricalDynamicsDSPBA_16fixed/8(Rphase_ohm)
  [SampleTime_s] -> ElectricalDynamicsDSPBA_16fixed/7(SampleTime_s)
  [iBeta_A_k_1] -> ElectricalDynamicsDSPBA_16fixed/6(iBeta_A_k_1)
  [iAlpha_A_k_1] -> ElectricalDynamicsDSPBA_16fixed/5(iAlpha_A_k_1)
  Mult/1 -> sfix16_En6/1  "ke*speed"
  [Ke_Vs_rad] -> Mult/2
  [dThetaMech_dt_rad_s] -> Mult/1
  Const2/1 -> Mux3/1
  iBeta_A_k_1/1 -> [iBeta_A_k_1]
  iAlpha_A_k_1/1 -> [iAlpha_A_k_1]
  dThetaMech_dt_rad_s/1 -> [dThetaMech_dt_rad_s]
  ThetaMech_one_turn/1 -> [ThetaMech_one_turn]
  inv_Lphase_1_H/1 -> [inv_Lphase_1_H]
  Rphase_ohm/1 -> [Rphase_ohm]
  Kt_Nm_A/1 -> [Kt_Nm_A]
  Ke_Vs_rad/1 -> [Ke_Vs_rad]
  SampleTime_s/1 -> [SampleTime_s]
  PolePairs_int/1 -> [PolePairs_int]
  Mux3/1 -> Inv_Park_16fixed/1(x_dq)
  Demux1/2 -> ElectricalDynamicsDSPBA_16fixed/2(vBemfBeta_V)  "vBemfBeta"
  Demux1/1 -> ElectricalDynamicsDSPBA_16fixed/1(vBemfAlpha_V)  "vBemfAlpha"
  Inv_Park_16fixed/1(x_AlphaBeta) -> Demux1/1
  [vAlpha_V] -> ElectricalDynamicsDSPBA_16fixed/3(vAlpha_V)
  [vBeta_V] -> ElectricalDynamicsDSPBA_16fixed/4(vBeta_V)
  Clarke_16fixed/1(xAlphaBeta) -> Demux5/1
  Demux5/2 -> [vBeta_V]
  Demux5/1 -> [vAlpha_V]  "vAlpha"
  Vabc_V/1 -> Clarke_16fixed/1(xabc)
  sfix16_En6/1 -> Mux3/2
  ElectricalDynamicsDSPBA_16fixed/4(iBeta_A_k) -> Mux7/2
  ElectricalDynamicsDSPBA_16fixed/3(iAlpha_A_k) -> Mux7/1
  sfix16_En14/1 -> T_Nm/1

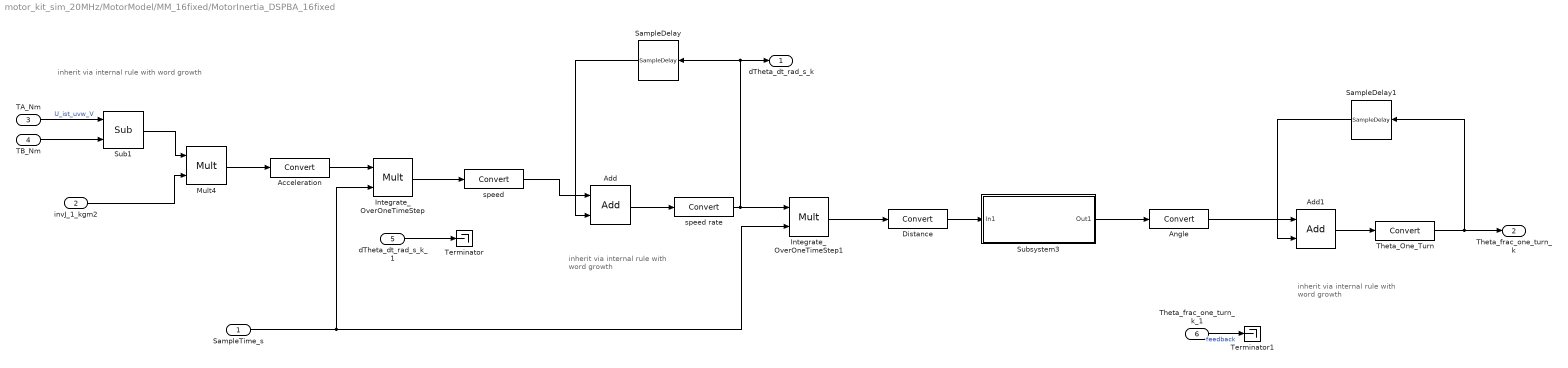
== system motor_kit_sim_20MHz/MotorModel/MM_16fixed/MotorInertia_DSPBA_16fixed ==
  note: inherit via internal rule with word growth
  note: inherit via internal rule
      | with word growth
  note: inherit via internal rule
      | with word growth
  SampleTime_s : Inport
  invJ_1_kgm2 : Inport  Port=2
  TA_Nm : Inport  Port=3
  TB_Nm : Inport  Port=4
  dTheta_dt_rad_s_k_1 : Inport  Port=5
  Theta_frac_one_turn_k_1 : Inport  Port=6
  Acceleration : DSPBAPrim/Convert  primtype=convert  nInputs=1  nOutputs=1  omode=Specify via dialog  otype=DataTypeAcceleration  scale=constScaleAcceleration  floatPrecision=float32_m23  rndmethod=Truncate  factor=1  satmethod=None  shift_vec=[0 1 2 -1]  value=round([0:255]/17)  inPortNames=[' '; ' ';]  outPortNames=[' '; 'c']  dspbaimage=dspba_prim_wide.svg  text=fprintf('convert');  clipdetect=off  advOptions=[]  version=20240711
  Add : DSPBAPrim/Add  primtype=add  nInputs=evalAionMaskParam(gcb,'value',1)  nOutputs=1  omode=Inherit via internal rule with word growth  otype=DataType  scale=constScaleSpeed  rndmethod=Unbiased  factor=1  satmethod=Symmetric  shift_vec=[0 1 2 -1]  value=2  inPortNames=[' '; ' ';]  outPortNames=[' ']  dspbaimage=dspba_prim.svg  text=fprintf('+');  genFPC=off  floatRounding=correct  advOptions=[]  version=20240716
  Add1 : DSPBAPrim/Add  primtype=add  nInputs=evalAionMaskParam(gcb,'value',1)  nOutputs=1  omode=Inherit via internal rule with word growth  otype=DataTypeUnsigned  scale=2^-16  rndmethod=Unbiased  factor=1  satmethod=Symmetric  shift_vec=[0 1 2 -1]  value=2  inPortNames=[' '; ' ';]  outPortNames=[' ']  dspbaimage=dspba_prim.svg  text=fprintf('+');  genFPC=off  floatRounding=correct  advOptions=[]  version=20240716
  Angle : DSPBAPrim/Convert  primtype=convert  nInputs=1  nOutputs=1  omode=Specify via dialog  otype=DataTypeTheta_OneTurn  scale=constScaleTheta_OneTurn  floatPrecision=float32_m23  rndmethod=Unbiased  factor=1  satmethod=None  shift_vec=[0 1 2 -1]  value=round([0:255]/17)  inPortNames=[' '; ' ';]  outPortNames=[' '; 'c']  dspbaimage=dspba_prim_wide.svg  text=fprintf('convert');  clipdetect=off  advOptions=[]  version=20240711
  Distance : DSPBAPrim/Convert  primtype=convert  nInputs=1  nOutputs=1  omode=Specify via dialog  otype=DataTypeDis  scale=constScaleDis  floatPrecision=float32_m23  rndmethod=Unbiased  factor=1  satmethod=None  shift_vec=[0 1 2 -1]  value=round([0:255]/17)  inPortNames=[' '; ' ';]  outPortNames=[' '; 'c']  dspbaimage=dspba_prim_wide.svg  text=fprintf('convert');  clipdetect=off  advOptions=[]  version=20240711
  Integrate_OverOneTimeStep : DSPBAPrim/Mult  primtype=mult  nInputs=2  nOutputs=1  omode=Inherit via internal rule  otype=DataType  scale=2^-12  floatPrecision=float32_m23  rndmethod=Unbiased  factor=1  satmethod=Symmetric  shift_vec=[0 1 2 -1]  value=0  inPortNames=[' '; ' ';]  outPortNames=[' ']  dspbaimage=dspba_prim.svg  text=fprintf('X');  floatRounding=correct  advOptions=[]  version=20240711
  Integrate_OverOneTimeStep1 : DSPBAPrim/Mult  primtype=mult  nInputs=2  nOutputs=1  omode=Inherit via internal rule  otype=sfix(32)  scale=2^-28  floatPrecision=float32_m23  rndmethod=Unbiased  factor=1  satmethod=Symmetric  shift_vec=[0 1 2 -1]  value=0  inPortNames=[' '; ' ';]  outPortNames=[' ']  dspbaimage=dspba_prim.svg  text=fprintf('X');  floatRounding=correct  advOptions=[]  version=20240711
  Mult4 : DSPBAPrim/Mult  primtype=mult  nInputs=2  nOutputs=1  omode=Inherit via internal rule  otype=DataTypeAcceleration  scale=2^0  floatPrecision=float32_m23  rndmethod=Unbiased  factor=1  satmethod=Symmetric  shift_vec=[0 1 2 -1]  value=0  inPortNames=[' '; ' ';]  outPortNames=[' ']  dspbaimage=dspba_prim.svg  text=fprintf('X');  floatRounding=correct  advOptions=[]  version=20240711
  SampleDelay : DSPBAPrim/SampleDelay  primtype=sampdelay  nInputs=1  nOutputs=1  omode=Inherit via internal rule  otype=sfix(16)  scale=2^-15  floatPrecision=float32_m23  rndmethod=Unbiased  factor=1  satmethod=Symmetric  shift_vec=[0 1 2 -1]  value=1  inPortNames=[' '; ' ';]  outPortNames=[' ']  dspbaimage=dspba_prim.svg  text=dpoly(1, eye(1,value+1), 'z')  flexible=off  slackgroup=0  augmented=0  version=20240711  advOptions=[]
  SampleDelay1 : DSPBAPrim/SampleDelay  primtype=sampdelay  nInputs=1  nOutputs=1  omode=Inherit via internal rule  otype=sfix(16)  scale=2^-15  floatPrecision=float32_m23  rndmethod=Unbiased  factor=1  satmethod=Symmetric  shift_vec=[0 1 2 -1]  value=1  inPortNames=[' '; ' ';]  outPortNames=[' ']  dspbaimage=dspba_prim.svg  text=dpoly(1, eye(1,value+1), 'z')  flexible=off  slackgroup=0  augmented=0  version=20240711  advOptions=[]
  Sub1 : DSPBAPrim/Sub  primtype=sub  nInputs=2  nOutputs=1  omode=Inherit via internal rule with word growth  otype=DataType  scale=constScaleTorque  rndmethod=Unbiased  factor=1  satmethod=Symmetric  shift_vec=[0 1 2 -1]  value=0  inPortNames=['+'; '-';]  outPortNames=[' ']  dspbaimage=dspba_prim.svg  text=fprintf('-');  floatRounding=correct  advOptions=[]  version=20240716
  Subsystem3 : Subsystem  mask{constVal=1/(2*pi)}
      mask prompts: constVal "Scaling phi elec"
      mask Display:
      | color('w');
      | set_param(gcb,'BackgroundColor','yellow');
      | fprintf('Scaling phi mech\n%s', num2str(constVal));
      | port_label('input',1, 'rad');
      | port_label('output',1,'turns');
  Terminator : Terminator
  Terminator1 : Terminator
  Theta_One_Turn : DSPBAPrim/Convert  primtype=convert  nInputs=1  nOutputs=1  omode=Specify via dialog  otype=DataTypeTheta_OneTurn  scale=constScaleTheta_OneTurn  floatPrecision=float32_m23  rndmethod=Unbiased  factor=1  satmethod=None  shift_vec=[0 1 2 -1]  value=round([0:255]/17)  inPortNames=[' '; ' ';]  outPortNames=[' '; 'c']  dspbaimage=dspba_prim_wide.svg  text=fprintf('convert');  clipdetect=off  advOptions=[]  version=20240711
  speed : DSPBAPrim/Convert  primtype=convert  nInputs=1  nOutputs=1  omode=Specify via dialog  otype=DataTypeSpeed  scale=constScaleSpeed  floatPrecision=float32_m23  rndmethod=Unbiased  factor=1  satmethod=None  shift_vec=[0 1 2 -1]  value=round([0:255]/17)  inPortNames=[' '; ' ';]  outPortNames=[' '; 'c']  dspbaimage=dspba_prim_wide.svg  text=fprintf('convert');  clipdetect=off  advOptions=[]  version=20240711
  speed rate : DSPBAPrim/Convert  primtype=convert  nInputs=1  nOutputs=1  omode=Specify via dialog  otype=DataTypeSpeedRate  scale=constScaleSpeedRate  floatPrecision=float32_m23  rndmethod=Unbiased  factor=1  satmethod=None  shift_vec=[0 1 2 -1]  value=round([0:255]/17)  inPortNames=[' '; ' ';]  outPortNames=[' '; 'c']  dspbaimage=dspba_prim_wide.svg  text=fprintf('convert');  clipdetect=off  advOptions=[]  version=20240711
  dTheta_dt_rad_s_k : Outport
  Theta_frac_one_turn_k : Outport  Port=2
  wires:
  Sub1/1 -> Mult4/1
  Add1/1 -> Theta_One_Turn/1
  Subsystem3/1(Out1) -> Angle/1
  SampleTime_s/1 -> Integrate_OverOneTimeStep/2, Integrate_OverOneTimeStep1/2
  TB_Nm/1 -> Sub1/2
  TA_Nm/1 -> Sub1/1  "U_ist_uvw_V"
  invJ_1_kgm2/1 -> Mult4/2
  Add/1 -> speed rate/1
  Integrate_OverOneTimeStep/1 -> speed/1
  Mult4/1 -> Acceleration/1
  Acceleration/1 -> Integrate_OverOneTimeStep/1
  speed/1 -> Add/1
  speed rate/1 -> dTheta_dt_rad_s_k/1, SampleDelay/1, Integrate_OverOneTimeStep1/1
  Distance/1 -> Subsystem3/1(In1)
  Integrate_OverOneTimeStep1/1 -> Distance/1
  Angle/1 -> Add1/1
  Theta_One_Turn/1 -> SampleDelay1/1, Theta_frac_one_turn_k/1
  SampleDelay/1 -> Add/2
  dTheta_dt_rad_s_k_1/1 -> Terminator/1
  SampleDelay1/1 -> Add1/2
  Theta_frac_one_turn_k_1/1 -> Terminator1/1  "feedback"

== system motor_kit_sim_20MHz/MotorModel/MM_16fixed/inverter ==
  note: If high transistor is connected, current is drawn from DC link.
      | Total DC link current is sum of currents flowing from DC link to motor terminals.
  note: Three motor terminal voltages.
  dc_link_V : Inport
  uvw_h : Inport  Port=2  OutDataTypeStr=boolean
  uvw_l : Inport  Port=3  OutDataTypeStr=boolean
  Iabc_A : Inport  Port=4
  Add3 : DSPBAPrim/Add  primtype=add  nInputs=evalAionMaskParam(gcb,'value',1)  nOutputs=1  omode=Specify via dialog  otype=sfix(19)  scale=2^-10  rndmethod=Unbiased  factor=1  satmethod=Symmetric  shift_vec=[0 1 2 -1]  value=3  inPortNames=[' '; ' ';]  outPortNames=[' ']  dspbaimage=dspba_prim.svg  text=fprintf('+');  genFPC=off  floatRounding=correct  advOptions=[]  version=20240716
  Constant1 : Constant  Value=0  OutDataTypeStr=fixdt(1,16,6)  SampleTime=DSPBASampleTime
  Demux1 : Demux  Outputs=3
  Demux4 : Demux  Outputs=3
  Mux : Mux  Inputs=3
  Mux{1..6} (6 alike) : DSPBAPrim/Mux  primtype=mux  nInputs=evalAionMaskParam(gcb,'value',1)+1  nOutputs=1  omode=Inherit via internal rule  otype=sfix(16)  scale=2^-15  rndmethod=Unbiased  factor=1  satmethod=Symmetric  shift_vec=[0 1 2 -1]  value=2  inPortNames=['s '; 'd0'; 'd1'; 'd2'; 'd3'; 'd4'; 'd5'; 'd6'; 'd7'; 'd8'; 'd9';]  outPortNames=[' ']  dspbaimage=dspba_prim_tall.svg  text=fprintf('%s', primtype);  version=20240715
  Terminator4 : Terminator
  Vabc_V : Outport
  dc_link_current_A : Outport  Port=2
  wires:
  Add3/1 -> dc_link_current_A/1
  Mux3/1 -> Mux/3
  uvw_h/1 -> Demux4/1
  Constant1/1 -> Mux6/2, Mux5/2, Mux4/2, Mux3/2, Mux2/2, Mux1/2
  Iabc_A/1 -> Demux1/1
  dc_link_V/1 -> Mux3/3, Mux2/3, Mux1/3
  uvw_l/1 -> Terminator4/1
  Demux4/1 -> Mux4/1, Mux1/1
  Demux4/2 -> Mux5/1, Mux2/1
  Demux4/3 -> Mux6/1, Mux3/1
  Mux/1 -> Vabc_V/1
  Mux1/1 -> Mux/1
  Mux2/1 -> Mux/2
  Mux4/1 -> Add3/1
  Mux5/1 -> Add3/2
  Mux6/1 -> Add3/3
  Demux1/1 -> Mux4/3
  Demux1/3 -> Mux6/3
  Demux1/2 -> Mux5/3
